simulink model "vcrdynamicsofthegears"  (R2020a)
settings: Solver=VariableStepAuto  StartTime=0.0  StopTime=10.0  RelTol=1e-3
undefined symbols (not defined in the file): g, m1, m1g, m2, magnitude, P, r1, rm, rm2, rtape, w1, x1, x2
settings Model: Creator=shanleymullen  LastModifiedBy=Aesop
settings DataIOCC: ReturnWorkspaceOutputs=off
settings DebuggingCC: ArithmeticOperatorsInVariantConditions=warning
settings SFSimCC: CustomCodeUndefinedFunction=UseInterfaceOnly

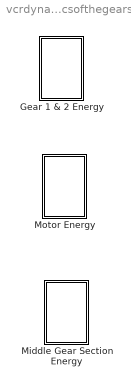
== system vcrdynamicsofthegears ==
  "Gear 1 & 2 Energy " : Subsystem
  Middle Gear Section Energy : Subsystem
  "Motor Energy " : Subsystem

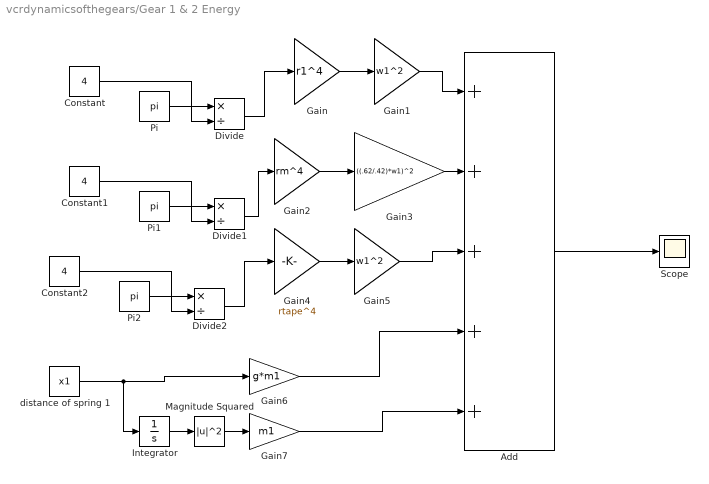
== system vcrdynamicsofthegears/Gear 1 & 2 Energy  ==
  Add : Sum  Inputs=+++++
  Constant : Constant  Value=4
  Constant1 : Constant  Value=4
  Constant2 : Constant  Value=4
  Divide : Product  Inputs=*/
  Divide1 : Product  Inputs=*/
  Divide2 : Product  Inputs=*/
  Gain : Gain  Gain=r1^4
  Gain1 : Gain  Gain=w1^2
  Gain2 : Gain  Gain=rm^4
  Gain3 : Gain  Gain=((.62/.42)*w1)^2
  Gain4 : Gain  Gain=rtape^4
  Gain5 : Gain  Gain=w1^2
  Gain6 : Gain  Gain=g*m1
  Gain7 : Gain  Gain=m1
  Integrator : Integrator
  Magnitude Squared : Math  Operator=magnitude^2  SignedPower=on  SaturateOnIntegerOverflow=on
  Pi : Constant  Value=pi  OutDataTypeStr=Inherit: Inherit via back propagation
  Pi1 : Constant  Value=pi  OutDataTypeStr=Inherit: Inherit via back propagation
  Pi2 : Constant  Value=pi  OutDataTypeStr=Inherit: Inherit via back propagation
  Scope : Scope
  "distance of spring 1 " : Constant  Value=x1
  wires:
  Gain6/1 -> Add/4
  Gain/1 -> Gain1/1
  Constant/1 -> Divide/2
  Gain5/1 -> Add/3
  Pi/1 -> Divide/1
  Divide1/1 -> Gain2/1
  Divide/1 -> Gain/1
  Gain2/1 -> Gain3/1
  "distance of spring 1 "/1 -> Integrator/1, Gain6/1
  Pi2/1 -> Divide2/1
  Pi1/1 -> Divide1/1
  Magnitude Squared/1 -> Gain7/1
  Constant1/1 -> Divide1/2
  Integrator/1 -> Magnitude Squared/1
  Gain1/1 -> Add/1
  Add/1 -> Scope/1
  Gain3/1 -> Add/2
  Gain7/1 -> Add/5
  Constant2/1 -> Divide2/2
  Gain4/1 -> Gain5/1
  Divide2/1 -> Gain4/1

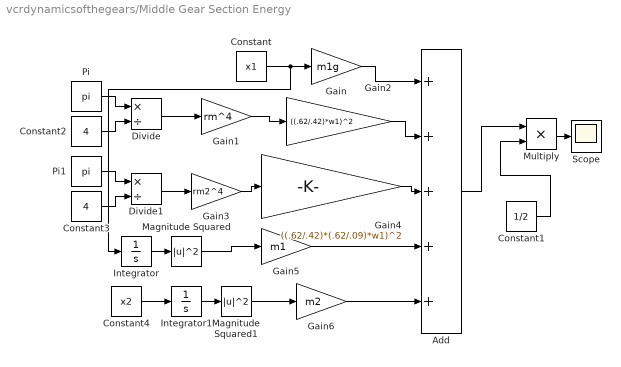
== system vcrdynamicsofthegears/Middle Gear Section Energy ==
  Add : Sum  Inputs=+++++
  Constant : Constant  Value=x1
  Constant1 : Constant  Value=1/2
  Constant2 : Constant  Value=4
  Constant3 : Constant  Value=4
  Constant4 : Constant  Value=x2
  Divide : Product  Inputs=*/
  Divide1 : Product  Inputs=*/
  Gain : Gain  Gain=m1g
  Gain1 : Gain  Gain=rm^4
  Gain2 : Gain  Gain=((.62/.42)*w1)^2
  Gain3 : Gain  Gain=rm2^4
  Gain4 : Gain  Gain=((.62/.42)*(.62/.09)*w1)^2
  Gain5 : Gain  Gain=m1
  Gain6 : Gain  Gain=m2
  Integrator : Integrator
  Integrator1 : Integrator
  Magnitude Squared : Math  Operator=magnitude^2  SignedPower=on  SaturateOnIntegerOverflow=on
  Magnitude Squared1 : Math  Operator=magnitude^2  SignedPower=on  SaturateOnIntegerOverflow=on
  Multiply : Product
  Pi : Constant  Value=pi  OutDataTypeStr=Inherit: Inherit via back propagation
  Pi1 : Constant  Value=pi  OutDataTypeStr=Inherit: Inherit via back propagation
  Scope : Scope
  wires:
  Constant/1 -> Integrator/1, Gain/1
  Integrator/1 -> Magnitude Squared/1
  Multiply/1 -> Scope/1
  Pi/1 -> Divide/1
  Magnitude Squared1/1 -> Gain6/1
  Gain4/1 -> Add/3
  Integrator1/1 -> Magnitude Squared1/1
  Constant4/1 -> Integrator1/1
  Magnitude Squared/1 -> Gain5/1
  Gain6/1 -> Add/5
  Add/1 -> Multiply/1
  Gain/1 -> Add/1
  Constant3/1 -> Divide1/2
  Constant1/1 -> Multiply/2
  Gain3/1 -> Gain4/1
  Constant2/1 -> Divide/2
  Divide/1 -> Gain1/1
  Gain1/1 -> Gain2/1
  Pi1/1 -> Divide1/1
  Gain2/1 -> Add/2
  Gain5/1 -> Add/4
  Divide1/1 -> Gain3/1

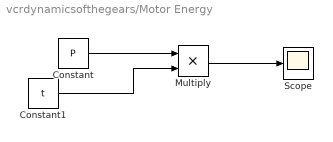
== system vcrdynamicsofthegears/Motor Energy  ==
  Constant : Constant  Value=P
  Constant1 : Constant  Value=t
  Multiply : Product
  Scope : Scope
  wires:
  Multiply/1 -> Scope/1
  Constant1/1 -> Multiply/2
  Constant/1 -> Multiply/1
